simulink model "ACT05"  (R2025b)
settings: Solver=VariableStepAuto  StartTime=0.0  StopTime=inf  RelTol=1e-3

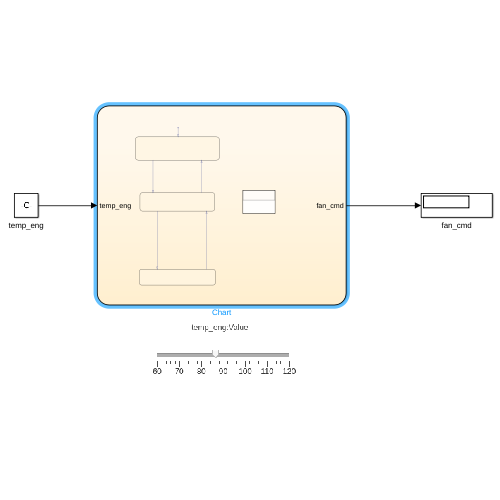
[thumbnail: Simulink's stored preview of the top-level diagram]
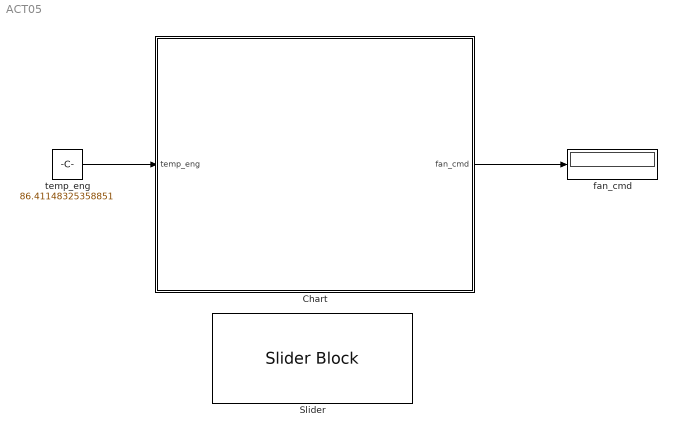
== system ACT05 ==
  Chart : Stateflow chart  TreatAsAtomicUnit=on
  Slider : SliderBlock  ScaleMin=60  ScaleMax=120
  fan_cmd : Display
  temp_eng : Constant  Value=86.41148325358851
  wires:
  temp_eng/1 -> Chart/1(temp_eng)
  Chart/1(fan_cmd) -> fan_cmd/1

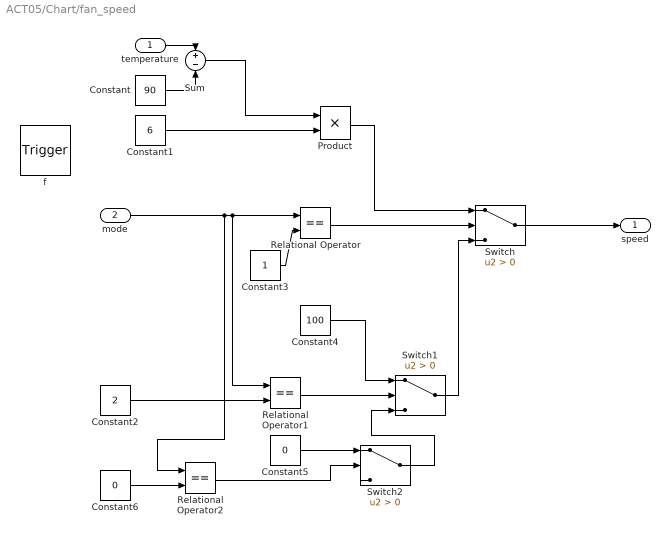
== system ACT05/Chart/fan_speed ==
  temperature : Inport  OutDataTypeStr=double  PortDimensions=1
  mode : Inport  Port=2  OutDataTypeStr=double  PortDimensions=1
  f : TriggerPort  TriggerType=function-call  VariantControl=(inherit)
      settings: CopyFcn=Stateflow.SLINSF.SimulinkMan.removeBlockPreDeleteFcn  PreDeleteFcn=Stateflow.SLINSF.SimulinkMan.unsafePredeleteFcn
  Constant : Constant  Value=90
  Constant1 : Constant  Value=6
  Constant2 : Constant  Value=2
  Constant3 : Constant
  Constant4 : Constant  Value=100
  Constant5 : Constant  Value=0
  Constant6 : Constant  Value=0
  Product : Product
  Relational Operator : RelationalOperator  Operator===  OutDataTypeStr=boolean  RndMeth=Simplest  InputSameDT=off
  Relational Operator1 : RelationalOperator  Operator===  OutDataTypeStr=boolean  RndMeth=Simplest  InputSameDT=off
  Relational Operator2 : RelationalOperator  Operator===  OutDataTypeStr=boolean  RndMeth=Simplest  InputSameDT=off
  Sum : Sum  Inputs=+-
  Switch : Switch  Criteria=u2 > Threshold  SaturateOnIntegerOverflow=off  InputSameDT=off
  Switch1 : Switch  Criteria=u2 > Threshold  SaturateOnIntegerOverflow=off  InputSameDT=off
  Switch2 : Switch  Criteria=u2 > Threshold  SaturateOnIntegerOverflow=off  InputSameDT=off
  speed : Outport  OutDataTypeStr=double  PortDimensions=1
  wires:
  temperature/1 -> Sum/1
  Constant/1 -> Sum/2
  Sum/1 -> Product/1
  Constant1/1 -> Product/2
  Relational Operator/1 -> Switch/2
  Product/1 -> Switch/1
  Switch/1 -> speed/1
  Constant3/1 -> Relational Operator/2
  mode/1 -> Relational Operator1/1, Relational Operator/1, Relational Operator2/1
  Relational Operator1/1 -> Switch1/2
  Constant2/1 -> Relational Operator1/2
  Constant4/1 -> Switch1/1
  Switch1/1 -> Switch/3
  Constant5/1 -> Switch2/1
  Relational Operator2/1 -> Switch2/2
  Constant6/1 -> Relational Operator2/2
  Switch2/1 -> Switch1/3

== stateflow chart ACT05/Chart ==
  state OFF
    entry:
    fan_cmd=fan_speed(temp_eng,0);
  state speed = fan_speed(temperature,mode) [function]
  state LOW
    during:
    fan_cmd=fan_speed(temp_eng,1);
  state HIGH
    entry:
    fan_cmd=fan_speed(temp_eng,2);
  (default) -> OFF
  OFF -> LOW : [temp_eng>=90]
  LOW -> OFF [order 2] : [temp_eng<88]
  LOW -> HIGH [order 1] : [temp_eng>=105]
  HIGH -> LOW : [temp_eng<103]
  data: temperature function_input double size=1; speed function_output double size=1; mode function_input double size=1; temp_eng input double size=1; fan_cmd output double size=1
